simulink model "tqdtqr_rebuild_V3"  (R2021b)
settings: Solver=VariableStepAuto  StartTime=0.0  StopTime=10.0  RelTol=1e-3
undefined symbols (not defined in the file): ATQD_AfterTqMinGain_X_Deg, ATQD_APSCreepBaseTqD_X_kph, ATQD_APSCreepBaseTqD_Y_Deg, ATQD_APSCreepBaseTqR_X_kph, ATQD_APSCreepBaseTqR_Y_Deg, ATQD_APSCreepIterm_X_kph, ATQD_APSCreepIterm_Y_kph, ATQD_APSCreepPterm_X_kph, ATQD_APSCreepPterm_Y_kph, ATQD_APSDecReq_X_kph, ATQD_APSDecReq_Y_mps2, ATQD_APSDecReqCMD_X_kph, ATQD_APSDecReqTs_X_pct, ATQD_APSDecTimeGain_X_Deg, ATQD_APSDecTimeGain_Y_s, ATQD_APSReqLowSpd_X_Deg, ATQD_AutoHoldReleaseBPS_X_Deg, ATQD_AWDLoadTrqnsGain_X_kg, ATQD_AWDLoadTrqnsGain_Y_pct, ATQD_BOSEnBPSPosn_X_kph, ATQD_BOSMap_X_rpm, ATQD_BOSMap_Y_pct, ATQD_CreepBaseTqD_X_kph, ATQD_CreepBaseTqD_Y_Deg, ATQD_CreepBaseTqR_X_kph, ATQD_CreepBaseTqR_Y_Deg, ATQD_CreepBPSDisPosn_X_Deg, ATQD_CreepBPSDisPosnR_X_Deg, ATQD_CreepBPSEnPosn_X_Deg, ATQD_CreepBPSEnPosnR_X_Deg, ATQD_CreepDeltaTq_X_kph, ATQD_CreepIterm_X_kph, ATQD_CreepIterm_Y_kph, ATQD_CreepItermMaxLimit_X_pct, ATQD_CreepPreloadTime_X_kph, ATQD_CreepPreloadTq_X_kph, ATQD_CreepPreloadTq_Y_s, ATQD_CreepProtTq_X_Deg, ATQD_CreepPterm_X_kph, ATQD_CreepPterm_Y_kph, ATQD_CreepRrTqSpRat_X_rpm, ATQD_CreepRrTqSpRat_Y_Nm, ATQD_CreepTargetSpdD_X_pct, ATQD_CreepTargetSpdR_X_pct, ATQD_CreepUpLimitTq_X_rpm, ATQD_DecIneOPDHoldEnDelay_X_Deg, ATQD_DecIneOPDHoldEnDelay_Y_bar, ATQD_ECOTqMapD_X_rpm, ATQD_ECOTqMapD_Y_pct, ATQD_EMTqMapD_X_rpm, ATQD_EMTqMapD_Y_pct, ATQD_EOPDTqMapDCon_X_rpm, ATQD_EOPDTqMapDCon_Y_Deg, ATQD_EstInitVehWeight_X_c, ATQD_FAfterTqCMDGain_X_rpm, ATQD_FAfterTqCMDGain_Y_pct, ATQD_ForceLowSpd_X_Deg, ATQD_ForcePLimitSpd_X_Deg, ATQD_FrLossMAPLowV_X_rpm, ATQD_FrLossMAPLowV_Y_Nm ... (+949)
libraries: simulink x235, hcu_lib x208, tqr x63, tqd x6
(part 10 of 37)

== system tqdtqr_rebuild_V3/Input_Convert/Main function/Front//Rear ramp parameters determine ==
  BSCPIn_outputs : Inport
  BSignalConvert_outputs : Inport  Port=2
  BFunction_outputs : Inport  Port=3
  BMain_outputs : Inport  Port=4
  VTQD_RollRegenEnable_flg : Inport  Port=5
  VTQD_TqSourceFr_enum : Inport  Port=6
  VTQD_EVDriveModeValid_flg : Inport  Port=7
  VTQD_PreLoadHold_flg : Inport  Port=8
  VTQD_CreepPrLoadEnable_flg : Inport  Port=9
  VTQD_PedAccTqEn_flg : Inport  Port=10
  VTQD_PreLoadPreEn_flg : Inport  Port=11
  VTQD_IVIRockModeEn_flg : Inport  Port=12
  VTQR_FrTqZeroTrans_enum : Inport  Port=13
  VTQD_RegenTqLimitEn_flg : Inport  Port=14
  VTQD_TqSourceRr_enum : Inport  Port=15
  VTQR_RrTqZeroTrans_enum : Inport  Port=16
  VTQD_FrZeroPointIncDec_Nm : Inport  Port=17
  VTQD_RrZeroPointIncDec_Nm : Inport  Port=18
  Bus Selector : BusSelector  OutputSignals=VTQD_ActAPSPosn_pct,VINP_VehSpeed_kph,VTQD_LimpHomeAct_flg,VVMC_ACCPedalOvrd_flg,VVMC_CCPedalOvrd_flg,VVMC_ActMaxSlideRate_pct,VTQD_RDCActive_enum,VVMC_MSAWhlTqActive_flg,VINP_FrPTCSActive_flg,VINP_IVISnowModeCmd_flg,VINP_VehicleType_enum,VINP_FrntAxlTrqReqDrv_Nm,VINP_RrPTCSActive_flg,VINP_RearAxlTrqReqDrv_Nm,VVMC_EstSlope_Deg,VINP_ACCVehHoldReq_flg,VPMM_DrivetrainSelect_enum,VVMC_ADASActive_flg
  Bus Selector1 : BusSelector  OutputSignals=VTQD_GearActualPosn_enum
  Bus Selector2 : BusSelector  OutputSignals=VTQD_TqTargetShaftSpd_rpm,VTQR_EVDriveMode_enum,VTQD_RegenMode_enum,VTQD_FrShaftSpd_rpm,VTQD_RrShaftSpd_rpm,VTQD_VehActSpd_kph
  Bus Selector3 : BusSelector  OutputSignals=VTQD_CoordWhlTqDemFr_Nm,VTQR_FEDUWhlTqReqSmoothDelay_Nm,VTQR_REDUWhlTqReqSmoothDelay_Nm,VTQR_RampREDUWhlTqReq_Nm,VTQR_RampFEDUWhlTqReq_Nm,VTQR_RrFirstOrderInpTq_Nm,VTQR_FrFirstOrderInpTq_Nm,VTQD_CoordWhlTqDemRr_Nm,VTQR_NoABSREDUWhlTqReq_Nm,VTQR_NoABSFEDUWhlTqReq_Nm
  Front First order filter input tau map and determination : Subsystem
  Front wheel rate limit determination : Subsystem
  Rear First order filter input tau map and determination : Subsystem
  Rear wheel rate limit determination1 : Subsystem
  VTQR_FrFirstOrderInpTs_c : Outport
  VTQR_FrRateLimitInc_Nm : Outport  Port=2
  VTQR_FrRateLimitDec_Nm : Outport  Port=3
  VTQR_RrFirstOrderInpTs_c : Outport  Port=4
  VTQR_RrRateLimitInc_Nm : Outport  Port=5
  VTQR_RrRateLimitDec_Nm : Outport  Port=6
  wires:
  Bus Selector2/1 -> [VTQD_TqTargetShaftSpd_rpm]  "<VTQD_TqTargetShaftSpd_rpm>"
  VTQD_RollRegenEnable_flg/1 -> [VTQD_RollRegenEnable_flg]
  BSCPIn_outputs/1 -> Bus Selector/1
  BSignalConvert_outputs/1 -> Bus Selector2/1
  Bus Selector2/2 -> [VTQR_EVDriveMode_enum]  "<VTQR_EVDriveMode_enum>"
  VTQD_TqSourceFr_enum/1 -> [VTQD_TqSourceFr_enum]
  Bus Selector/1 -> [VDHP_ActAPSPosn_pct]  "<VTQD_ActAPSPosn_pct>"
  Bus Selector/2 -> [VINP_VehSpeed_kph]  "<VINP_VehSpeed_kph>"
  Bus Selector/3 -> [VTQD_LimpHomeAct_flg]  "<VTQD_LimpHomeAct_flg>"
  VTQD_EVDriveModeValid_flg/1 -> [VTQD_EVDriveModeValid_flg]
  Bus Selector2/3 -> [VTQD_RegenMode_enum]  "<VTQD_RegenMode_enum>"
  Bus Selector/4 -> [VVMC_ACCPedalOvrd_flg]  "<VVMC_ACCPedalOvrd_flg>"
  Bus Selector/5 -> [VVMC_CCPedalOvrd_flg]  "<VVMC_CCPedalOvrd_flg>"
  VTQD_PreLoadHold_flg/1 -> [VTQD_PreLoadHold_flg]
  VTQD_CreepPrLoadEnable_flg/1 -> [VTQD_CreepPrLoadEnable_flg]
  Bus Selector/6 -> [VVMC_ActMaxSlideRate_pct]  "<VVMC_ActMaxSlideRate_pct>"
  Bus Selector/7 -> [VTQD_RDCActive_enum]  "<VTQD_RDCActive_enum>"
  VTQD_PedAccTqEn_flg/1 -> [VTQD_PedAccTqEn_flg]
  VTQD_PreLoadPreEn_flg/1 -> [VTQD_PreLoadPreEn_flg]
  Bus Selector/8 -> [VVMC_MSAWhlTqActive_flg]  "<VVMC_MSAWhlTqActive_flg>"
  Bus Selector/9 -> [VINP_FrPTCSActive_flg]  "<VINP_FrPTCSActive_flg>"
  Bus Selector/10 -> [VINP_IVISnowModeCmd_flg]  "<VINP_IVISnowModeCmd_flg>"
  VTQD_IVIRockModeEn_flg/1 -> [VTQD_IVIRockModeEn_flg]
  Bus Selector/11 -> [VINP_VehicleType_enum]  "<VINP_VehicleType_enum>"
  BMain_outputs/1 -> Bus Selector3/1
  Bus Selector3/1 -> [VTQD_CoordWhlTqDemFr_Nm]  "<VTQD_CoordWhlTqDemFr_Nm>"
  Bus Selector/12 -> [VINP_FrntAxlTrqReqDrv_Nm]  "<VINP_FrntAxlTrqReqDrv_Nm>"
  [VVMC_CCPedalOvrd_flg] -> Front First order filter input tau map and determination/12(VVMC_CCPedalOvrd_flg)
  [VTQD_LimpHomeAct_flg] -> Front First order filter input tau map and determination/8(VTQD_LimpHomeAct_flg)
  [VINP_VehSpeed_kph] -> Front First order filter input tau map and determination/7(VINP_VehSpeed_kph)
  [VDHP_ActAPSPosn_pct] -> Front First order filter input tau map and determination/6(VDHP_ActAPSPosn_pct)
  [VTQR_RampFEDUWhlTqReq_Nm] -> Front First order filter input tau map and determination/18(VTQR_RampFEDUWhlTqReq_Nm)
  [VTQD_PreLoadHold_flg] -> Front First order filter input tau map and determination/13(VTQD_PreLoadHold_flg)
  [VTQR_NoABSFEDUWhlTqReq_Nm] -> Front First order filter input tau map and determination/17(VTQR_NoABSFEDUWhlTqReq_Nm)
  [VVMC_MSAWhlTqActive_flg] -> Front First order filter input tau map and determination/22(VVMC_MSAWhlTqActive_flg)
  [VTQD_EVDriveModeValid_flg] -> Front First order filter input tau map and determination/9(VTQD_EVDriveModeValid_flg)
  [VVMC_ActMaxSlideRate_pct] -> Front First order filter input tau map and determination/14(VVMC_ActMaxSlideRate_pct)
  [VINP_FrPTCSActive_flg] -> Front First order filter input tau map and determination/23(VINP_FrPTCSActive_flg)
  [VTQR_EVDriveMode_enum] -> Front First order filter input tau map and determination/2(VTQR_EVDriveMode_enum)
  [VTQD_CoordWhlTqDemFr_Nm] -> Front First order filter input tau map and determination/27(VTQD_CoordWhlTqDemFr_Nm)
  [VINP_FrntAxlTrqReqDrv_Nm] -> Front First order filter input tau map and determination/28(VINP_FrntAxlTrqReqDrv_Nm)
  [VVMC_ACCPedalOvrd_flg] -> Front First order filter input tau map and determination/11(VVMC_ACCPedalOvrd_flg)
  [VTQD_RDCActive_enum] -> Front First order filter input tau map and determination/16(VTQD_RDCActive_enum)
  [VTQR_FEDUWhlTqReqSmoothDelay_Nm] -> Front First order filter input tau map and determination/5(VTQR_FEDUWhlTqReqSmoothDelay_Nm)
  [VTQD_RegenMode_enum] -> Front First order filter input tau map and determination/10(VTQD_RegenMode_enum)
  Front First order filter input tau map and determination/1(VTQR_FrFirstOrderInpTs_c) -> [VTQR_FrFirstOrderInpTs_c]
  [VTQD_PedAccTqEn_flg] -> Front First order filter input tau map and determination/20(VTQD_PedAccTqEn_flg)
  [VTQD_IVIRockModeEn_flg] -> Front First order filter input tau map and determination/25(VTQD_IVIRockModeEn_flg)
  [VTQD_TqSourceFr_enum] -> Front First order filter input tau map and determination/4(VTQD_TqSourceFr_enum)
  [VTQR_FrFirstOrderInpTq_Nm] -> Front First order filter input tau map and determination/19(VTQR_FrFirstOrderInpTq_Nm)
  [VINP_IVISnowModeCmd_flg] -> Front First order filter input tau map and determination/24(VINP_IVISnowModeCmd_flg)
  [VTQD_PreLoadPreEn_flg] -> Front First order filter input tau map and determination/21(VTQD_PreLoadPreEn_flg)
  [VTQD_RollRegenEnable_flg] -> Front First order filter input tau map and determination/3(VTQD_RollRegenEnable_flg)
  [VINP_VehicleType_enum] -> Front First order filter input tau map and determination/26(VINP_VehicleType_enum)
  [VTQD_CreepPrLoadEnable_flg] -> Front First order filter input tau map and determination/15(VTQD_CreepPrLoadEnable_flg)
  [VTQD_TqTargetShaftSpd_rpm] -> Front First order filter input tau map and determination/1(VTQD_TqTargetShaftSpd_rpm)
  [VTQR_FrTqZeroTrans_enum] -> Front wheel rate limit determination/1(VTQR_FrTqZeroTrans_enum)
  [VTQD_GearActualPosn_enum] -> Front wheel rate limit determination/23(VTQD_GearActualPosn_enum)
  [VTQD_EVDriveModeValid_flg] -> Front wheel rate limit determination/8(VTQD_EVDriveModeValid_flg)
  [VTQD_TqTargetShaftSpd_rpm] -> Front wheel rate limit determination/3(VTQD_TqTargetShaftSpd_rpm)
  [VTQD_RDCActive_enum] -> Front wheel rate limit determination/14(VTQD_RDCActive_enum)
  [VTQR_FrFirstOrderInpTq_Nm] -> Front wheel rate limit determination/18(VTQR_FrFirstOrderInpTq_Nm)
  [VTQR_RampFEDUWhlTqReq_Nm] -> Front wheel rate limit determination/17(VTQR_RampFEDUWhlTqReq_Nm)
  [VINP_FrntAxlTrqReqDrv_Nm] -> Front wheel rate limit determination/29(VINP_FrntAxlTrqReqDrv_Nm)
  [VTQD_TqSourceFr_enum] -> Front wheel rate limit determination/2(VTQD_TqSourceFr_enum)
  [VTQD_CoordWhlTqDemFr_Nm] -> Front wheel rate limit determination/28(VTQD_CoordWhlTqDemFr_Nm)
  [VTQD_CreepPrLoadEnable_flg] -> Front wheel rate limit determination/12(VTQD_CreepPrLoadEnable_flg)
  [VTQD_RegenTqLimitEn_flg] -> Front wheel rate limit determination/13(VTQD_RegenTqLimitEn_flg)
  [VTQD_RegenMode_enum] -> Front wheel rate limit determination/9(VTQD_RegenMode_enum)
  [VTQR_EVDriveMode_enum] -> Front wheel rate limit determination/5(VTQR_EVDriveMode_enum)
  Front wheel rate limit determination/2(VTQR_FrRateLimitDec_Nm) -> [VTQR_FrRateLimitDec_Nm]
  [VINP_IVISnowModeCmd_flg] -> Front wheel rate limit determination/24(VINP_IVISnowModeCmd_flg)
  [VINP_VehicleType_enum] -> Front wheel rate limit determination/27(VINP_VehicleType_enum)
  [VINP_FrPTCSActive_flg] -> Front wheel rate limit determination/22(VINP_FrPTCSActive_flg)
  [VTQR_NoABSFEDUWhlTqReq_Nm] -> Front wheel rate limit determination/16(VTQR_NoABSFEDUWhlTqReq_Nm)
  [VDHP_ActAPSPosn_pct] -> Front wheel rate limit determination/6(VDHP_ActAPSPosn_pct)
  [VTQD_PreLoadPreEn_flg] -> Front wheel rate limit determination/15(VTQD_PreLoadPreEn_flg)
  [VTQD_PedAccTqEn_flg] -> Front wheel rate limit determination/20(VTQD_PedAccTqEn_flg)
  [VVMC_ActMaxSlideRate_pct] -> Front wheel rate limit determination/19(VVMC_ActMaxSlideRate_pct)
  [VTQD_IVIRockModeEn_flg] -> Front wheel rate limit determination/25(VTQD_IVIRockModeEn_flg)
  [VVMC_MSAWhlTqActive_flg] -> Front wheel rate limit determination/21(VVMC_MSAWhlTqActive_flg)
  [VVMC_CCPedalOvrd_flg] -> Front wheel rate limit determination/11(VVMC_CCPedalOvrd_flg)
  [VTQR_FEDUWhlTqReqSmoothDelay_Nm] -> Front wheel rate limit determination/7(VTQR_FEDUWhlTqReqSmoothDelay_Nm)
  [VTQD_FrShaftSpd_rpm] -> Front wheel rate limit determination/26(VTQD_FrShaftSpd_rpm)
  Front wheel rate limit determination/1(VTQR_FrRateLimitInc_Nm) -> [VTQR_FrRateLimitInc_Nm]
  [VTQD_LimpHomeAct_flg] -> Front wheel rate limit determination/4(VTQD_LimpHomeAct_flg)
  [VVMC_ACCPedalOvrd_flg] -> Front wheel rate limit determination/10(VVMC_ACCPedalOvrd_flg)
  VTQR_FrTqZeroTrans_enum/1 -> [VTQR_FrTqZeroTrans_enum]
  VTQD_RegenTqLimitEn_flg/1 -> [VTQD_RegenTqLimitEn_flg]
  BFunction_outputs/1 -> Bus Selector1/1
  Bus Selector1/1 -> [VTQD_GearActualPosn_enum]  "<VTQD_GearActualPosn_enum>"
  Bus Selector2/4 -> [VTQD_FrShaftSpd_rpm]  "<VTQD_FrShaftSpd_rpm>"
  [VTQD_LimpHomeAct_flg] -> Rear First order filter input tau map and determination/8(VTQD_LimpHomeAct_flg)
  [VINP_VehSpeed_kph] -> Rear First order filter input tau map and determination/7(VINP_VehSpeed_kph)
  [VDHP_ActAPSPosn_pct] -> Rear First order filter input tau map and determination/6(VDHP_ActAPSPosn_pct)
  [VTQD_RollRegenEnable_flg] -> Rear First order filter input tau map and determination/3(VTQD_RollRegenEnable_flg)
  [VTQD_TqTargetShaftSpd_rpm] -> Rear First order filter input tau map and determination/1(VTQD_TqTargetShaftSpd_rpm)
  [VTQR_NoABSREDUWhlTqReq_Nm] -> Rear First order filter input tau map and determination/17(VTQR_NoABSREDUWhlTqReq_Nm)
  [VTQD_IVIRockModeEn_flg] -> Rear First order filter input tau map and determination/25(VTQD_IVIRockModeEn_flg)
  [VINP_VehicleType_enum] -> Rear First order filter input tau map and determination/26(VINP_VehicleType_enum)
  [VTQD_RDCActive_enum] -> Rear First order filter input tau map and determination/16(VTQD_RDCActive_enum)
  [VTQD_EVDriveModeValid_flg] -> Rear First order filter input tau map and determination/9(VTQD_EVDriveModeValid_flg)
  [VTQD_CreepPrLoadEnable_flg] -> Rear First order filter input tau map and determination/15(VTQD_CreepPrLoadEnable_flg)
  [VTQR_EVDriveMode_enum] -> Rear First order filter input tau map and determination/2(VTQR_EVDriveMode_enum)
  [VTQD_CoordWhlTqDemRr_Nm] -> Rear First order filter input tau map and determination/27(VTQD_CoordWhlTqDemRr_Nm)
  [VTQD_PedAccTqEn_flg] -> Rear First order filter input tau map and determination/20(VTQD_PedAccTqEn_flg)
  [VTQD_PreLoadPreEn_flg] -> Rear First order filter input tau map and determination/21(VTQD_PreLoadPreEn_flg)
  [VINP_RearAxlTrqReqDrv_Nm] -> Rear First order filter input tau map and determination/28(VINP_RearAxlTrqReqDrv_Nm)
  [VINP_RrPTCSActive_flg] -> Rear First order filter input tau map and determination/23(VINP_RrPTCSActive_flg)
  [VTQR_REDUWhlTqReqSmoothDelay_Nm] -> Rear First order filter input tau map and determination/5(VTQR_REDUWhlTqReqSmooth_Nm)
  [VTQR_RampREDUWhlTqReq_Nm] -> Rear First order filter input tau map and determination/18(VTQR_RampREDUWhlTqReq_Nm)
  [VVMC_ActMaxSlideRate_pct] -> Rear First order filter input tau map and determination/14(VVMC_ActMaxSlideRate_pct)
  [VVMC_CCPedalOvrd_flg] -> Rear First order filter input tau map and determination/12(VVMC_CCPedalOvrd_flg)
  [VTQD_PreLoadHold_flg] -> Rear First order filter input tau map and determination/13(VTQD_PreLoadHold_flg)
  [VVMC_MSAWhlTqActive_flg] -> Rear First order filter input tau map and determination/22(VVMC_MSAWhlTqActive_flg)
  [VTQR_RrFirstOrderInpTq_Nm] -> Rear First order filter input tau map and determination/19(VTQR_RrFirstOrderInpTq_Nm)
  [VINP_IVISnowModeCmd_flg] -> Rear First order filter input tau map and determination/24(VINP_IVISnowModeCmd_flg)
  [VTQD_TqSourceRr_enum] -> Rear First order filter input tau map and determination/4(VTQD_TqSourceRr_enum)
  [VTQD_RegenMode_enum] -> Rear First order filter input tau map and determination/10(VTQD_RegenMode_enum)
  [VVMC_ACCPedalOvrd_flg] -> Rear First order filter input tau map and determination/11(VVMC_ACCPedalOvrd_flg)
  VTQD_TqSourceRr_enum/1 -> [VTQD_TqSourceRr_enum]
  Bus Selector/13 -> [VINP_RrPTCSActive_flg]  "<VINP_RrPTCSActive_flg>"
  Bus Selector/14 -> [VINP_RearAxlTrqReqDrv_Nm]  "<VINP_RearAxlTrqReqDrv_Nm>"
  [VTQD_TqTargetShaftSpd_rpm] -> Rear wheel rate limit determination1/3(VTQD_TqTargetShaftSpd_rpm)
  [VTQD_RDCActive_enum] -> Rear wheel rate limit determination1/14(VTQD_RDCActive_enum)
  [VVMC_CCPedalOvrd_flg] -> Rear wheel rate limit determination1/11(VVMC_CCPedalOvrd_flg)
  [VTQD_EVDriveModeValid_flg] -> Rear wheel rate limit determination1/8(VTQD_EVDriveModeValid_flg)
  [VTQR_REDUWhlTqReqSmoothDelay_Nm] -> Rear wheel rate limit determination1/7(VTQR_REDUWhlTqReqSmoothDelay_Nm)
  [VTQR_EVDriveMode_enum] -> Rear wheel rate limit determination1/5(VTQR_EVDriveMode_enum)
  [VTQR_RrTqZeroTrans_enum] -> Rear wheel rate limit determination1/1(VTQR_RrTqZeroTrans_enum)
  [VTQR_NoABSREDUWhlTqReq_Nm] -> Rear wheel rate limit determination1/16(VTQR_NoABSREDUWhlTqReq_Nm)
  [VVMC_ADASActive_flg] -> Rear wheel rate limit determination1/31(VVMC_ADASActive_flg)
  [VINP_RearAxlTrqReqDrv_Nm] -> Rear wheel rate limit determination1/34(VINP_RearAxlTrqReqDrv_Nm)
  [VTQD_RrShaftSpd_rpm] -> Rear wheel rate limit determination1/26(VTQD_RrShaftSpd_rpm)
  [VTQD_VehActSpd_kph] -> Rear wheel rate limit determination1/28(VTQD_VehActSpd_kph)
  [VTQD_CreepPrLoadEnable_flg] -> Rear wheel rate limit determination1/12(VTQD_CreepPrLoadEnable_flg)
  [VVMC_ACCPedalOvrd_flg] -> Rear wheel rate limit determination1/10(VVMC_ACCPedalOvrd_flg)
  [VVMC_EstSlope_Deg] -> Rear wheel rate limit determination1/27(VVMC_EstSlope_Deg)
  [VINP_RrPTCSActive_flg] -> Rear wheel rate limit determination1/22(VINP_RrPTCSActive_flg)
  [VTQD_RegenTqLimitEn_flg] -> Rear wheel rate limit determination1/13(VTQD_RegenTqLimitEn_flg)
  [VTQR_RampREDUWhlTqReq_Nm] -> Rear wheel rate limit determination1/17(VTQR_RampREDUWhlTqReq_Nm)
  [VINP_VehicleType_enum] -> Rear wheel rate limit determination1/32(VINP_VehicleType_enum)
  Rear wheel rate limit determination1/2(VTQR_RrRateLimitDec_Nm) -> [VTQR_RrRateLimitDec_Nm]
  [VINP_ACCVehHoldReq_flg] -> Rear wheel rate limit determination1/29(VINP_ACCVehHoldReq_flg)
  [VTQD_GearActualPosn_enum] -> Rear wheel rate limit determination1/23(VTQD_GearActualPosn_enum)
  [VTQD_LimpHomeAct_flg] -> Rear wheel rate limit determination1/4(VTQD_LimpHomeAct_flg)
  [VTQD_IVIRockModeEn_flg] -> Rear wheel rate limit determination1/25(VTQD_IVIRockModeEn_flg)
  [VTQD_CoordWhlTqDemRr_Nm] -> Rear wheel rate limit determination1/33(VTQD_CoordWhlTqDemRr_Nm)
  [VPMM_DriveTrainSelect_enum] -> Rear wheel rate limit determination1/30(VPMM_DriveTrainSelect_enum)
  [VINP_IVISnowModeCmd_flg] -> Rear wheel rate limit determination1/24(VINP_IVISnowModeCmd_flg)
  [VVMC_MSAWhlTqActive_flg] -> Rear wheel rate limit determination1/21(VVMC_MSAWhlTqActive_flg)
  [VTQD_TqSourceRr_enum] -> Rear wheel rate limit determination1/2(VTQD_TqSourceRr_enum)
  [VTQD_PedAccTqEn_flg] -> Rear wheel rate limit determination1/20(VTQD_PedAccTqEn_flg)
  [VTQD_PreLoadPreEn_flg] -> Rear wheel rate limit determination1/15(VTQD_PreLoadPreEn_flg)
  [VTQD_RegenMode_enum] -> Rear wheel rate limit determination1/9(VTQD_RegenMode_enum)
  [VVMC_ActMaxSlideRate_pct] -> Rear wheel rate limit determination1/19(VVMC_ActMaxSlideRate_pct)
  Rear wheel rate limit determination1/1(VTQR_RrRateLimitInc_Nm) -> [VTQR_RrRateLimitInc_Nm]
  [VTQR_RrFirstOrderInpTq_Nm] -> Rear wheel rate limit determination1/18(VTQR_RrFirstOrderInpTq_Nm)
  [VDHP_ActAPSPosn_pct] -> Rear wheel rate limit determination1/6(VDHP_ActAPSPosn_pct)
  VTQR_RrTqZeroTrans_enum/1 -> [VTQR_RrTqZeroTrans_enum]
  Bus Selector2/5 -> [VTQD_RrShaftSpd_rpm]  "<VTQD_RrShaftSpd_rpm>"
  Bus Selector/15 -> [VVMC_EstSlope_Deg]  "<VVMC_EstSlope_Deg>"
  Bus Selector2/6 -> [VTQD_VehActSpd_kph]  "<VTQD_VehActSpd_kph>"
  Bus Selector/16 -> [VINP_ACCVehHoldReq_flg]  "<VINP_ACCVehHoldReq_flg>"
  Bus Selector/17 -> [VPMM_DriveTrainSelect_enum]  "<VPMM_DrivetrainSelect_enum>"
  Bus Selector/18 -> [VVMC_ADASActive_flg]  "<VVMC_ADASActive_flg>"
  [VTQR_FrFirstOrderInpTs_c] -> VTQR_FrFirstOrderInpTs_c/1
  [VTQR_FrRateLimitInc_Nm] -> VTQR_FrRateLimitInc_Nm/1
  [VTQR_FrRateLimitDec_Nm] -> VTQR_FrRateLimitDec_Nm/1
  [VTQR_RrFirstOrderInpTs_c] -> VTQR_RrFirstOrderInpTs_c/1
  [VTQR_RrRateLimitInc_Nm] -> VTQR_RrRateLimitInc_Nm/1
  [VTQR_RrRateLimitDec_Nm] -> VTQR_RrRateLimitDec_Nm/1
  Bus Selector3/2 -> [VTQR_FEDUWhlTqReqSmoothDelay_Nm]  "<VTQR_FEDUWhlTqReqSmoothDelay_Nm>"
  Bus Selector3/3 -> [VTQR_REDUWhlTqReqSmoothDelay_Nm]  "<VTQR_REDUWhlTqReqSmoothDelay_Nm>"
  Bus Selector3/4 -> [VTQR_RampREDUWhlTqReq_Nm]  "<VTQR_RampREDUWhlTqReq_Nm>"
  Bus Selector3/5 -> [VTQR_RampFEDUWhlTqReq_Nm]  "<VTQR_RampFEDUWhlTqReq_Nm>"
  Bus Selector3/6 -> [VTQR_RrFirstOrderInpTq_Nm]  "<VTQR_RrFirstOrderInpTq_Nm>"
  Bus Selector3/7 -> [VTQR_FrFirstOrderInpTq_Nm]  "<VTQR_FrFirstOrderInpTq_Nm>"
  Bus Selector3/8 -> [VTQD_CoordWhlTqDemRr_Nm]  "<VTQD_CoordWhlTqDemRr_Nm>"
  Bus Selector3/9 -> [VTQR_NoABSREDUWhlTqReq_Nm]  "<VTQR_NoABSREDUWhlTqReq_Nm>"
  Bus Selector3/10 -> [VTQR_NoABSFEDUWhlTqReq_Nm]  "<VTQR_NoABSFEDUWhlTqReq_Nm>"
  VTQD_FrZeroPointIncDec_Nm/1 -> [VTQD_FrZeroPointIncDec_Nm]
  VTQD_RrZeroPointIncDec_Nm/1 -> [VTQD_RrZeroPointIncDec_Nm]
  [VTQD_FrZeroPointIncDec_Nm] -> Front wheel rate limit determination/30(VTQD_FrZeroPointIncDec_Nm)
  [VTQD_RrZeroPointIncDec_Nm] -> Rear wheel rate limit determination1/35(VTQD_RrZeroPointIncDec_Nm)
  Rear First order filter input tau map and determination/1(VTQR_RrFirstOrderInpTs_c) -> [VTQR_RrFirstOrderInpTs_c]  "VTQR_RrFirstOrderInpTs_c"
  [VVMC_EstSlope_Deg] -> Front First order filter input tau map and determination/29(VVMC_EstSlope_Deg)
  [VVMC_EstSlope_Deg] -> Rear First order filter input tau map and determination/29(VVMC_EstSlope_Deg)
  [VVMC_EstSlope_Deg] -> Front wheel rate limit determination/31(VVMC_EstSlope_Deg)

== system tqdtqr_rebuild_V3/Input_Convert/Main function/Front//Rear wheel torque different function ==
  note: Rear
  note: Front
  BSCPIn_outputs : Inport
  BSignalConvert_outputs : Inport  Port=2
  AND{,1..3} (4 alike) : Logic  AllPortsSameDT=off  OutDataTypeStr=boolean
  Abs : Abs
  Abs1 : Abs
  Add1 : Sum  Inputs=+-
  Add2 : Sum  Inputs=+-
  Bus Selector : BusSelector  OutputSignals=task_time_s,VINP_LFRawWhlSpeed_kph,VINP_RFRawWhlSpeed_kph,VINP_ABSActive_flg,VINP_FrPTCSActive_flg,VINP_LRRawWhlSpeed_kph,VINP_RRRawWhlSpeed_kph,VINP_RrPTCSActive_flg
  Bus Selector1 : BusSelector  OutputSignals=VTQD_LowIdleAccPedal_flg
  Delay{,1..3} (4 alike) : Delay  DelayLength=1  InitialCondition=single(0)
      settings: AttributesFormatString=%<InitialCondition>
  Divide{,1..3} (4 alike) : Product  Inputs=***/
  FirstOrderFilter : hcu_lib/Basic_Blocks/FirstOrderFilter
  FirstOrderFilter1 : hcu_lib/Basic_Blocks/FirstOrderFilter
  MTQR_FShaftSpdTqLimCoe_Y_c : Lookup_n-D  NumberOfTableDimensions=1  BreakpointsForDimension1=ATQR_FShaftSpdTqLimCoe_X_rpm  Table=MTQR_FShaftSpdTqLimCoe_Y_c  InternalRulePriority=Speed  RndMeth=Simplest  InputSameDT=on
  MTQR_FTimerTqLimCoe_Y_c : Lookup_n-D  NumberOfTableDimensions=1  BreakpointsForDimension1=ATQR_FTimerTqLimCoe_X_s  Table=MTQR_FTimerTqLimCoe_Y_c  InternalRulePriority=Speed  RndMeth=Simplest  InputSameDT=on
  MTQR_RShaftSpdTqLimCoe_Y_c : Lookup_n-D  NumberOfTableDimensions=1  BreakpointsForDimension1=ATQR_RShaftSpdTqLimCoe_X_rpm  Table=MTQR_RShaftSpdTqLimCoe_Y_c  InternalRulePriority=Speed  RndMeth=Simplest  InputSameDT=on
  MTQR_RTimerTqLimCoe_Y_c : Lookup_n-D  NumberOfTableDimensions=1  BreakpointsForDimension1=ATQR_RTimerTqLimCoe_X_s  Table=MTQR_RTimerTqLimCoe_Y_c  InternalRulePriority=Speed  RndMeth=Simplest  InputSameDT=on
  Min{1..4} (4 alike) : MinMax  Inputs=2
  NOT{,1..5} (6 alike) : Logic  Operator=NOT  AllPortsSameDT=off  OutDataTypeStr=boolean
  OR{1..4} (4 alike) : Logic  Operator=OR  AllPortsSameDT=off  OutDataTypeStr=boolean
  RegenLV_inc{1,6,10,15} (4 alike) : Constant  Value=KPH2MPS  OutDataTypeStr=single
  RegenLV_inc{2,7,11,16} (4 alike) : Constant  Value=KTQD_TireRadius_m  OutDataTypeStr=single
  RegenLV_inc12 : Constant  Value=KTQR_FShaftSpdDevTs_c  OutDataTypeStr=single
  RegenLV_inc13 : Constant  Value=KTQR_StartTimerShaftDev_rpm  OutDataTypeStr=single
  RegenLV_inc14 : Constant  Value=KTQR_ShaftSpdDevTime_s  OutDataTypeStr=single
  RegenLV_inc{17,19,23,25} (4 alike) : Constant  Value=ONE_FLOAT  OutDataTypeStr=single
  RegenLV_inc18 : Constant  Value=KTQR_FShaftSpdTqCoeLimLow_c  OutDataTypeStr=single
  RegenLV_inc20 : Constant  Value=KTQR_FTimerTqCoeLimLow_c  OutDataTypeStr=single
  RegenLV_inc{8..9,21..22} (4 alike) : Constant  Value=RADPS2RPM  OutDataTypeStr=single
  RegenLV_inc24 : Constant  Value=KTQR_RShaftSpdTqCoeLimLow_c  OutDataTypeStr=single
  RegenLV_inc26 : Constant  Value=KTQR_RTimerTqCoeLimLow_c  OutDataTypeStr=single
  RegenLV_inc3 : Constant  Value=KTQR_RShaftSpdDevTs_c  OutDataTypeStr=single
  RegenLV_inc4 : Constant  Value=KTQR_StartTimerShaftDev_rpm  OutDataTypeStr=single
  RegenLV_inc5 : Constant  Value=KTQR_ShaftSpdDevTime_s  OutDataTypeStr=single
  Relational Operator : RelationalOperator  Operator=>  OutDataTypeStr=boolean  RndMeth=Simplest
  Relational Operator{1..2,4..5} (4 alike) : RelationalOperator  Operator=<=  OutDataTypeStr=boolean  RndMeth=Simplest
  Relational Operator3 : RelationalOperator  Operator=>  OutDataTypeStr=boolean  RndMeth=Simplest
  SR_Latch{,1..3} (4 alike) : hcu_lib/Basic_Blocks/SR_Latch
  Switch{1..8} (8 alike) : Switch  Criteria=u2 ~= 0
      settings: AttributesFormatString=%<Criteria>
  Timer : hcu_lib/Basic_Blocks/Timer
  Timer1 : hcu_lib/Basic_Blocks/Timer
  VTQR_FShaftSpdTqLimCoe_c : Outport
  VTQR_FTimerTqLimCoe_c : Outport  Port=2
  VTQR_RShaftSpdTqLimCoe_c : Outport  Port=3
  VTQR_RTimerTqLimCoe_c : Outport  Port=4
  VTQR_FShaftSpdTqLimLow_flg : Outport  Port=5
  VTQR_FTimerTqLimLow_flg : Outport  Port=6
  VTQR_RShaftSpdTqLimLow_flg : Outport  Port=7
  VTQR_RTimerTqLimLow_flg : Outport  Port=8
  wires:
  [VTQR_LFWheelShaftSpd_rpm] -> Add1/1
  Abs/1 -> [VTQR_ActFShaftSpdDev_rpm]  "VTQR_ActFShaftSpdDev_rpm"
  RegenLV_inc14/1 -> Timer/4
  Add1/1 -> FirstOrderFilter/1  "VTQR_FWheelShaftSpdDev_rpm"
  [VINP_RFRawWhlSpeed_kph] -> Divide1/1
  Timer/1 -> [VTQR_FShaftSpdDevTime_s]  "VTQR_FShaftSpdDevTime_s"
  Divide1/1 -> [VTQR_RFWheelShaftSpd_rpm]  "VTQR_RFWheelShaftSpd_rpm"
  Divide/1 -> [VTQR_LFWheelShaftSpd_rpm]  "VTQR_LFWheelShaftSpd_rpm"
  [task_time_s] -> Timer/3
  RegenLV_inc7/1 -> Divide1/4
  RegenLV_inc8/1 -> Divide1/3
  RegenLV_inc6/1 -> Divide1/2
  RegenLV_inc9/1 -> Divide/3
  RegenLV_inc13/1 -> Relational Operator/2
  Relational Operator/1 -> Timer/1, NOT/1
  RegenLV_inc11/1 -> Divide/4
  [VTQR_ActFShaftSpdDev_rpm] -> Relational Operator/1
  [VTQR_RFWheelShaftSpd_rpm] -> Add1/2
  RegenLV_inc10/1 -> Divide/2
  NOT/1 -> Timer/2
  [task_time_s] -> FirstOrderFilter/2
  [VINP_LFRawWhlSpeed_kph] -> Divide/1
  RegenLV_inc12/1 -> FirstOrderFilter/3
  FirstOrderFilter/1 -> Abs/1
  [VTQR_FTimerTqLimLow_flg] -> Switch5/2
  Switch2/1 -> [VTQR_InitFShaftSpdTqLimCoe_c]  "VTQR_InitFShaftSpdTqLimCoe_c"
  RegenLV_inc20/1 -> Relational Operator2/2
  [VTQD_LowIdleAccPedal_flg] -> AND1/2
  Switch5/1 -> [VTQR_FTimerTqLimCoe_c], Delay1/1  "VTQR_FTimerTqLimCoe_c"
  Min2/1 -> Switch5/1
  SR_Latch1/1 -> [VTQR_FTimerTqLimLow_flg]  "VTQR_FTimerTqLimLow_flg"
  Delay1/1 -> Min2/1
  [VTQR_InitFTimerTqLimCoe_c] -> Switch5/3
  SR_Latch/1 -> [VTQR_FShaftSpdTqLimLow_flg]  "VTQR_FShaftSpdTqLimLow_flg"
  Min1/1 -> Switch4/1
  [VTQR_InitFShaftSpdTqLimCoe_c] -> Switch4/3
  AND1/1 -> SR_Latch1/2
  Relational Operator2/1 -> SR_Latch1/1, NOT2/1
  [VTQR_FShaftSpdTqLimLow_flg] -> Switch4/2
  [VTQR_InitFShaftSpdTqLimCoe_c] -> Relational Operator1/1
  NOT2/1 -> AND1/1
  [VTQR_InitFTimerTqLimCoe_c] -> Relational Operator2/1
  OR2/1 -> Switch3/2
  [VINP_FrPTCSActive_flg] -> OR2/2
  RegenLV_inc19/1 -> Switch3/1
  [VINP_ABSActive_flg] -> OR2/1
  [VTQD_LowIdleAccPedal_flg] -> AND/2
  Relational Operator1/1 -> NOT1/1, SR_Latch/1
  MTQR_FShaftSpdTqLimCoe_Y_c/1 -> Switch2/3
  RegenLV_inc17/1 -> Switch2/1
  AND/1 -> SR_Latch/2
  RegenLV_inc18/1 -> Relational Operator1/2
  [VINP_FrPTCSActive_flg] -> OR1/2
  Switch3/1 -> [VTQR_InitFTimerTqLimCoe_c]  "VTQR_InitFTimerTqLimCoe_c"
  [VTQR_ActFShaftSpdDev_rpm] -> MTQR_FShaftSpdTqLimCoe_Y_c/1
  NOT1/1 -> AND/1
  [VTQR_InitFTimerTqLimCoe_c] -> Min2/2
  [VTQR_FShaftSpdDevTime_s] -> MTQR_FTimerTqLimCoe_Y_c/1
  [VINP_ABSActive_flg] -> OR1/1
  OR1/1 -> Switch2/2
  MTQR_FTimerTqLimCoe_Y_c/1 -> Switch3/3
  [VTQR_InitFShaftSpdTqLimCoe_c] -> Min1/2
  Delay/1 -> Min1/1
  Switch4/1 -> Delay/1, [VTQR_FShaftSpdTqLimCoe_c]  "VTQR_FShaftSpdTqLimCoe_c"
  [VTQR_RRWheelShaftSpd_rpm] -> Add2/2
  [VINP_RRRawWhlSpeed_kph] -> Divide3/1
  NOT3/1 -> Timer1/2
  RegenLV_inc2/1 -> Divide2/4
  RegenLV_inc5/1 -> Timer1/4
  [task_time_s] -> Timer1/3
  Timer1/1 -> [VTQR_RShaftSpdDevTime_s]  "VTQR_RShaftSpdDevTime_s"
  [VINP_LRRawWhlSpeed_kph] -> Divide2/1
  [VTQR_ActRShaftSpdDev_rpm] -> Relational Operator3/1
  Abs1/1 -> [VTQR_ActRShaftSpdDev_rpm]  "VTQR_ActRShaftSpdDev_rpm"
  Relational Operator3/1 -> Timer1/1, NOT3/1
  Divide3/1 -> [VTQR_RRWheelShaftSpd_rpm]  "VTQR_RRWheelShaftSpd_rpm"
  RegenLV_inc4/1 -> Relational Operator3/2
  [task_time_s] -> FirstOrderFilter1/2
  FirstOrderFilter1/1 -> Abs1/1
  [VTQR_LRWheelShaftSpd_rpm] -> Add2/1
  Add2/1 -> FirstOrderFilter1/1  "VTQR_RWheelShaftSpdDev_rpm"
  RegenLV_inc21/1 -> Divide3/3
  RegenLV_inc15/1 -> Divide3/2
  Divide2/1 -> [VTQR_LRWheelShaftSpd_rpm]  "VTQR_LRWheelShaftSpd_rpm"
  RegenLV_inc3/1 -> FirstOrderFilter1/3
  RegenLV_inc16/1 -> Divide3/4
  RegenLV_inc22/1 -> Divide2/3
  RegenLV_inc1/1 -> Divide2/2
  [VINP_RrPTCSActive_flg] -> OR4/2
  Delay2/1 -> Min3/1
  [VTQR_InitRShaftSpdTqLimCoe_c] -> Switch7/3
  NOT5/1 -> AND3/1
  [VTQD_LowIdleAccPedal_flg] -> AND3/2
  [VINP_RrPTCSActive_flg] -> OR3/2
  [VTQR_RTimerTqLimLow_flg] -> Switch8/2
  Switch6/1 -> [VTQR_InitRTimerTqLimCoe_c]  "VTQR_InitRTimerTqLimCoe_c"
  Switch7/1 -> [VTQR_RShaftSpdTqLimCoe_c], Delay2/1  "VTQR_RShaftSpdTqLimCoe_c"
  [VTQR_RShaftSpdTqLimLow_flg] -> Switch7/2
  [VTQD_LowIdleAccPedal_flg] -> AND2/2
  AND2/1 -> SR_Latch2/2
  [VINP_ABSActive_flg] -> OR4/1
  SR_Latch3/1 -> [VTQR_RTimerTqLimLow_flg]  "VTQR_RTimerTqLimLow_flg"
  [VTQR_InitRTimerTqLimCoe_c] -> Switch8/3
  Relational Operator4/1 -> NOT4/1, SR_Latch2/1
  [VTQR_InitRShaftSpdTqLimCoe_c] -> Min3/2
  RegenLV_inc24/1 -> Relational Operator4/2
  Switch1/1 -> [VTQR_InitRShaftSpdTqLimCoe_c]  "VTQR_InitRShaftSpdTqLimCoe_c"
  Delay3/1 -> Min4/1
  Min3/1 -> Switch7/1
  MTQR_RTimerTqLimCoe_Y_c/1 -> Switch6/3
  Switch8/1 -> [VTQR_RTimerTqLimCoe_c], Delay3/1  "VTQR_RTimerTqLimCoe_c"
  [VTQR_RShaftSpdDevTime_s] -> MTQR_RTimerTqLimCoe_Y_c/1
  [VTQR_ActRShaftSpdDev_rpm] -> MTQR_RShaftSpdTqLimCoe_Y_c/1
  [VTQR_InitRShaftSpdTqLimCoe_c] -> Relational Operator4/1
  [VTQR_InitRTimerTqLimCoe_c] -> Min4/2
  [VTQR_InitRTimerTqLimCoe_c] -> Relational Operator5/1
  AND3/1 -> SR_Latch3/2
  RegenLV_inc26/1 -> Relational Operator5/2
  Min4/1 -> Switch8/1
  MTQR_RShaftSpdTqLimCoe_Y_c/1 -> Switch1/3
  RegenLV_inc23/1 -> Switch1/1
  [VINP_ABSActive_flg] -> OR3/1
  RegenLV_inc25/1 -> Switch6/1
  SR_Latch2/1 -> [VTQR_RShaftSpdTqLimLow_flg]  "VTQR_RShaftSpdTqLimLow_flg"
  OR3/1 -> Switch1/2
  OR4/1 -> Switch6/2
  Relational Operator5/1 -> SR_Latch3/1, NOT5/1
  NOT4/1 -> AND2/1
  BSCPIn_outputs/1 -> Bus Selector/1
  BSignalConvert_outputs/1 -> Bus Selector1/1
  Bus Selector/2 -> [VINP_LFRawWhlSpeed_kph]  "<VINP_LFRawWhlSpeed_kph>"
  Bus Selector/1 -> [task_time_s]  "<task_time_s>"
  Bus Selector/3 -> [VINP_RFRawWhlSpeed_kph]  "<VINP_RFRawWhlSpeed_kph>"
  Bus Selector/4 -> [VINP_ABSActive_flg]  "<VINP_ABSActive_flg>"
  Bus Selector/5 -> [VINP_FrPTCSActive_flg]  "<VINP_FrPTCSActive_flg>"
  Bus Selector1/1 -> [VTQD_LowIdleAccPedal_flg]  "<VTQD_LowIdleAccPedal_flg>"
  Bus Selector/6 -> [VINP_LRRawWhlSpeed_kph]  "<VINP_LRRawWhlSpeed_kph>"
  Bus Selector/7 -> [VINP_RRRawWhlSpeed_kph]  "<VINP_RRRawWhlSpeed_kph>"
  Bus Selector/8 -> [VINP_RrPTCSActive_flg]  "<VINP_RrPTCSActive_flg>"
  [VTQR_FShaftSpdTqLimCoe_c] -> VTQR_FShaftSpdTqLimCoe_c/1
  [VTQR_FTimerTqLimCoe_c] -> VTQR_FTimerTqLimCoe_c/1
  [VTQR_RShaftSpdTqLimCoe_c] -> VTQR_RShaftSpdTqLimCoe_c/1
  [VTQR_RTimerTqLimCoe_c] -> VTQR_RTimerTqLimCoe_c/1
  [VTQR_FShaftSpdTqLimLow_flg] -> VTQR_FShaftSpdTqLimLow_flg/1
  [VTQR_FTimerTqLimLow_flg] -> VTQR_FTimerTqLimLow_flg/1
  [VTQR_RShaftSpdTqLimLow_flg] -> VTQR_RShaftSpdTqLimLow_flg/1
  [VTQR_RTimerTqLimLow_flg] -> VTQR_RTimerTqLimLow_flg/1

== system tqdtqr_rebuild_V3/Input_Convert/Main function/Front//Rear wheel torque limitation determine function ==
  BSCPIn_outputs : Inport
  BMain_outputs : Inport  Port=2
  VTQR_FShaftSpdTqLimCoe_c : Inport  Port=3
  VTQR_FTimerTqLimCoe_c : Inport  Port=4
  VTQR_RShaftSpdTqLimCoe_c : Inport  Port=5
  VTQR_RTimerTqLimCoe_c : Inport  Port=6
  Add : Sum  Inputs=++-
  Add1 : Sum  Inputs=++-
  Bus Selector : BusSelector  OutputSignals=VTQD_AfterAvailableTqDemFr_Nm,VTQD_AfterAvailableTqDemRr_Nm,VTQR_REDUWhlTqReqSmoothDelay_Nm,VTQR_FEDUWhlTqReqSmoothDelay_Nm
  Bus Selector1 : BusSelector  OutputSignals=VPMM_DrivetrainSelect_enum
  Equal : RelationalOperator  Operator===  OutDataTypeStr=boolean  RndMeth=Simplest
  Equal1 : RelationalOperator  Operator===  OutDataTypeStr=boolean  RndMeth=Simplest
  Min : MinMax  Inputs=2
  Min1 : MinMax  Inputs=2
  OR : Logic  AllPortsSameDT=off  OutDataTypeStr=boolean
  OR1 : Logic  AllPortsSameDT=off  OutDataTypeStr=boolean
  Product{,1..3} (4 alike) : Product  Inputs=3
  RegenLV_inc1 : Constant  Value=KTQR_FinalFEDUTrqLowLim_Nm  OutDataTypeStr=single
  RegenLV_inc10 : Constant  Value=KTQR_FinalREDUTrqLowLim_Nm  OutDataTypeStr=single
  RegenLV_inc11 : Constant  Value=KTQR_RgnShaftSpdProtSW_flg  OutDataTypeStr=single
  RegenLV_inc12 : Constant  Value=KTQR_FinalREDUTrqLowLim_Nm  OutDataTypeStr=single
  RegenLV_inc15 : Constant  Value=KTQR_FinalFEDUTrqLowLim_Nm  OutDataTypeStr=single
  RegenLV_inc16 : Constant  Value=KTQR_RgnShaftSpdProtSW_flg  OutDataTypeStr=single
  RegenLV_inc2 : Constant  Value=KTQR_FinalFEDUTrqUpLim_Nm  OutDataTypeStr=single
  RegenLV_inc3 : Constant  Value=KTQR_FEDUTrqUpLimSW_flg  OutDataTypeStr=single
  RegenLV_inc4 : Constant  Value=KTQR_FinalFEDUTrqUpLim_Nm  OutDataTypeStr=single
  RegenLV_inc5 : Constant  Value=ENUM_DRIVETRAIN_AWD  OutDataTypeStr=single
  RegenLV_inc6 : Constant  Value=KTQR_FinalREDUTrqUpLim_Nm  OutDataTypeStr=single
  RegenLV_inc7 : Constant  Value=KTQR_REDUTrqUpLimSW_flg  OutDataTypeStr=single
  RegenLV_inc8 : Constant  Value=KTQR_FinalREDUTrqUpLim_Nm  OutDataTypeStr=single
  RegenLV_inc9 : Constant  Value=ENUM_DRIVETRAIN_AWD  OutDataTypeStr=single
  Switch{,1..3} (4 alike) : Switch  Criteria=u2 ~= 0
      settings: AttributesFormatString=%<Criteria>
  VTQR_ActFEDUTrqUpLim_Nm : Outport
  VTQR_ActFEDUTrqLowLim_Nm : Outport  Port=2
  VTQR_ActREDUTrqUpLim_Nm : Outport  Port=3
  VTQR_ActREDUTrqLowLim_Nm : Outport  Port=4
  wires:
  Min/1 -> Switch1/1  "VTQR_CoorFEDUTrqUpLim_Nm"
  Add/1 -> Min/1  "VTQR_CalFEDUTrqUpLim_Nm"
  [VTQR_FShaftSpdTqLimCoe_c] -> Product/2
  Switch1/1 -> Product/1
  RegenLV_inc5/1 -> Equal/2
  [VTQR_FTimerTqLimCoe_c] -> Product/3
  RegenLV_inc2/1 -> Min/2
  [VTQD_AfterAvailableTqDemRr_Nm] -> Add/2
  [VPMM_DriveTrainSelect_enum] -> Equal/1
  [VTQD_AfterAvailableTqDemFr_Nm] -> Add/1
  Equal/1 -> OR/1
  [VTQR_REDUWhlTqReqSmoothDelay_Nm] -> Add/3
  RegenLV_inc3/1 -> OR/2
  RegenLV_inc4/1 -> Switch1/3
  OR/1 -> Switch1/2
  Product/1 -> [VTQR_ActFEDUTrqUpLim_Nm]  "VTQR_ActFEDUTrqUpLim_Nm"
  Switch/1 -> [VTQR_ActFEDUTrqLowLim_Nm]  "VTQR_ActFEDUTrqLowLim_Nm"
  [VTQR_FTimerTqLimCoe_c] -> Product1/2
  RegenLV_inc15/1 -> Product1/3
  Product1/1 -> Switch/1
  [VTQR_FShaftSpdTqLimCoe_c] -> Product1/1
  RegenLV_inc1/1 -> Switch/3
  RegenLV_inc16/1 -> Switch/2
  Min1/1 -> Switch2/1  "VTQR_CoorREDUTrqUpLim_Nm"
  [VTQR_RShaftSpdTqLimCoe_c] -> Product2/2
  RegenLV_inc9/1 -> Equal1/2
  [VPMM_DriveTrainSelect_enum] -> Equal1/1
  RegenLV_inc7/1 -> OR1/2
  [VTQR_RTimerTqLimCoe_c] -> Product2/3
  Switch2/1 -> Product2/1
  Product2/1 -> [VTQR_ActREDUTrqUpLim_Nm]  "VTQR_ActREDUTrqUpLim_Nm"
  OR1/1 -> Switch2/2
  [VTQR_FEDUWhlTqReqSmoothDelay_Nm] -> Add1/3
  RegenLV_inc8/1 -> Min1/2
  Equal1/1 -> OR1/1
  [VTQD_AfterAvailableTqDemRr_Nm] -> Add1/2
  Add1/1 -> Min1/1  "VTQR_CalREDUTrqUpLim_Nm"
  [VTQD_AfterAvailableTqDemFr_Nm] -> Add1/1
  RegenLV_inc6/1 -> Switch2/3
  RegenLV_inc11/1 -> Switch3/2
  [VTQR_RTimerTqLimCoe_c] -> Product3/2
  Product3/1 -> Switch3/1
  [VTQR_RShaftSpdTqLimCoe_c] -> Product3/1
  RegenLV_inc10/1 -> Product3/3
  RegenLV_inc12/1 -> Switch3/3
  Switch3/1 -> [VTQR_ActREDUTrqLowLim_Nm]  "VTQR_ActREDUTrqLowLim_Nm"
  VTQR_FShaftSpdTqLimCoe_c/1 -> [VTQR_FShaftSpdTqLimCoe_c]
  VTQR_FTimerTqLimCoe_c/1 -> [VTQR_FTimerTqLimCoe_c]
  VTQR_RShaftSpdTqLimCoe_c/1 -> [VTQR_RShaftSpdTqLimCoe_c]
  VTQR_RTimerTqLimCoe_c/1 -> [VTQR_RTimerTqLimCoe_c]
  BMain_outputs/1 -> Bus Selector/1
  Bus Selector/1 -> [VTQD_AfterAvailableTqDemFr_Nm]  "<VTQD_AfterAvailableTqDemFr_Nm>"
  Bus Selector/2 -> [VTQD_AfterAvailableTqDemRr_Nm]  "<VTQD_AfterAvailableTqDemRr_Nm>"
  BSCPIn_outputs/1 -> Bus Selector1/1
  Bus Selector1/1 -> [VPMM_DriveTrainSelect_enum]  "<VPMM_DrivetrainSelect_enum>"
  [VTQR_ActFEDUTrqUpLim_Nm] -> VTQR_ActFEDUTrqUpLim_Nm/1
  [VTQR_ActFEDUTrqLowLim_Nm] -> VTQR_ActFEDUTrqLowLim_Nm/1
  [VTQR_ActREDUTrqUpLim_Nm] -> VTQR_ActREDUTrqUpLim_Nm/1
  [VTQR_ActREDUTrqLowLim_Nm] -> VTQR_ActREDUTrqLowLim_Nm/1
  Bus Selector/3 -> [VTQR_REDUWhlTqReqSmoothDelay_Nm]  "<VTQR_REDUWhlTqReqSmoothDelay_Nm>"
  Bus Selector/4 -> [VTQR_FEDUWhlTqReqSmoothDelay_Nm]  "<VTQR_FEDUWhlTqReqSmoothDelay_Nm>"
